simulink model "Solar_Batt_H2_PowerFlow_Solution_Lithium"  (R2023b)
settings: Solver=ode8  StartTime=0.0  StopTime=17520  FixedStep=1  RelTol=1e-3
values from neighbouring files (symbols this model uses):
  k1 = 0.6705    [main.m]
  n_batt = 40    [main.m]
  nb_set_solar_panel = 20    [main.m]
settings Model: Creator=pacel
settings DebuggingCC: UnconnectedInputMsg=warning  UnconnectedOutputMsg=warning  UnconnectedLineMsg=warning
settings ModelReferenceCC: EnableRefExpFcnMdlSchedulingChecks=on
settings RTWCC: DLArmComputeVersion=19.05

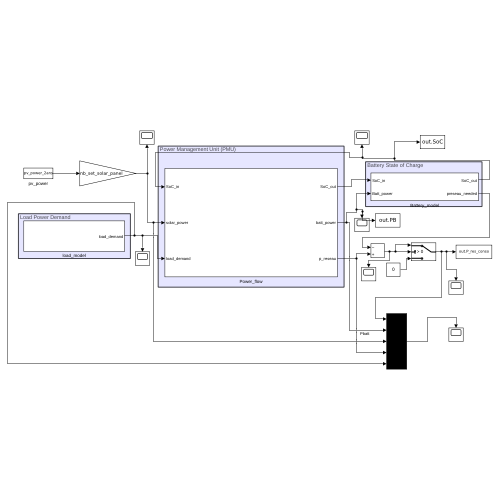
[thumbnail: Simulink's stored preview of the top-level diagram]
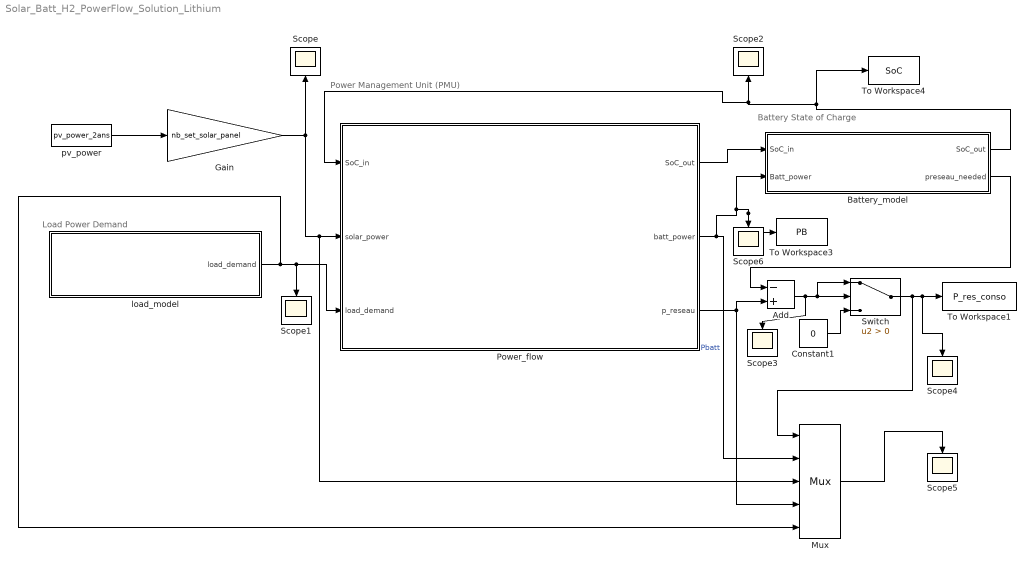
== system Solar_Batt_H2_PowerFlow_Solution_Lithium ==
  note: Load Power Demand
  note: Battery State of Charge
  note: Power Management Unit (PMU)
  Add : Sum  Inputs=-+
  Battery_model : Subsystem
  Constant1 : Constant  Value=0
  Gain : Gain  Gain=nb_set_solar_panel
  Mux : Mux  Inputs=5
  Power_flow : Subsystem
  Scope{,1..6} (7 alike) : Scope
  Switch : Switch  Criteria=u2 > Threshold  SaturateOnIntegerOverflow=off  InputSameDT=off
  To Workspace1 : ToWorkspace  VariableName=P_res_conso  SaveFormat=Timeseries  SampleTime=-1
  To Workspace3 : ToWorkspace  VariableName=PB  SaveFormat=Timeseries  SampleTime=-1
  To Workspace4 : ToWorkspace  VariableName=SoC  SaveFormat=Timeseries  SampleTime=-1
  load_model : Subsystem
  pv_power : FromWorkspace  VariableName=pv_power_2ans  OutDataTypeStr=double  SampleTime=1
  wires:
  Power_flow/2(batt_power) -> Battery_model/2(Batt_power), Scope6/1, To Workspace3/1, Mux/2  "Pbatt"
  load_model/1(load_demand) -> Mux/5, Scope1/1, Power_flow/3(load_demand)
  pv_power/1 -> Gain/1
  Battery_model/1(SoC_out) -> To Workspace4/1, Scope2/1, Power_flow/1(SoC_in)
  Power_flow/1(SoC_out) -> Battery_model/1(SoC_in)
  Gain/1 -> Scope/1, Mux/3, Power_flow/2(solar_power)
  Constant1/1 -> Switch/3
  Switch/1 -> Mux/1, Scope4/1, To Workspace1/1
  Mux/1 -> Scope5/1
  Power_flow/3(p_reseau) -> Mux/4, Add/2
  Battery_model/2(preseau_needed) -> Add/1
  Add/1 -> Scope3/1, Switch/2, Switch/1

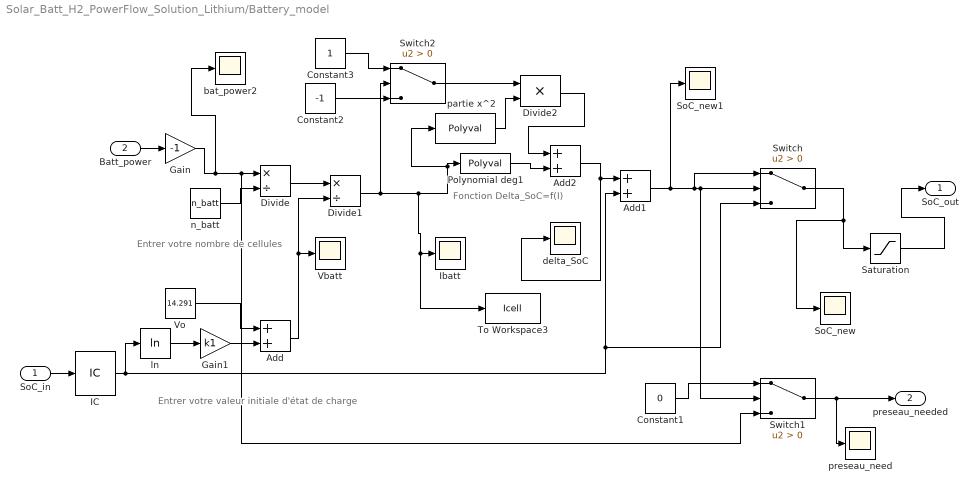
== system Solar_Batt_H2_PowerFlow_Solution_Lithium/Battery_model ==
  note: Entrer votre valeur initiale d'état de charge
  note: Entrer votre nombre de cellules
  note: Fonction Delta_SoC=f(I)
  SoC_in : Inport
  Batt_power : Inport  Port=2
  Add : Sum
  Add1 : Sum
  Add2 : Sum
  Constant1 : Constant  Value=0
  Constant2 : Constant  Value=-1
  Constant3 : Constant
  Divide : Product  Inputs=*/
  Divide1 : Product  Inputs=*/
  Divide2 : Product  Inputs=**
  Gain : Gain  Gain=-1
  Gain1 : Gain  Gain=k1
  IC : InitialCondition  Value=0.5
  Ibatt : Scope
  Polynomial deg1 : Polyval  Coefs=[ +0.01, -0.004 ]
  Saturation : Saturate  UpperLimit=0.95  LowerLimit=0.05
  SoC_new : Scope
  SoC_new1 : Scope
  Switch : Switch  Criteria=u2 > Threshold  SaturateOnIntegerOverflow=off  InputSameDT=off
  Switch1 : Switch  Criteria=u2 > Threshold  SaturateOnIntegerOverflow=off  InputSameDT=off
  Switch2 : Switch  Criteria=u2 > Threshold  SaturateOnIntegerOverflow=off  InputSameDT=off
  To Workspace3 : ToWorkspace  VariableName=Icell  SaveFormat=Timeseries  SampleTime=-1
  Vbatt : Scope
  Vo : Constant  Value=14.291
  bat_power2 : Scope
  delta_SoC : Scope
  ln : Math  Operator=log
  n_batt : Constant  Value=n_batt
  partie x^2 : Polyval  Coefs=[ 0, 0, 0]
  preseau_need : Scope
  SoC_out : Outport
  preseau_needed : Outport  Port=2
  wires:
  Saturation/1 -> SoC_out/1
  Batt_power/1 -> Gain/1
  Add/1 -> Divide1/2, Vbatt/1
  SoC_in/1 -> IC/1
  Vo/1 -> Add/1
  Divide1/1 -> Switch2/2, partie x^2/1, Polynomial deg1/1, To Workspace3/1, Ibatt/1
  Divide/1 -> Divide1/1
  Polynomial deg1/1 -> Add2/2
  n_batt/1 -> Divide/2
  Gain/1 -> bat_power2/1, Switch1/3, Divide/1
  Gain1/1 -> Add/2
  Switch/1 -> SoC_new/1, Saturation/1
  Add1/1 -> SoC_new1/1, Switch1/2, Switch/2, Switch/1
  Constant1/1 -> Switch1/1
  Switch1/1 -> preseau_need/1, preseau_needed/1
  Constant3/1 -> Switch2/1
  Constant2/1 -> Switch2/3
  Switch2/1 -> Divide2/1
  partie x^2/1 -> Divide2/2
  Divide2/1 -> Add2/1
  Add2/1 -> delta_SoC/1, Add1/1
  IC/1 -> ln/1, Switch/3, Add1/2
  ln/1 -> Gain1/1

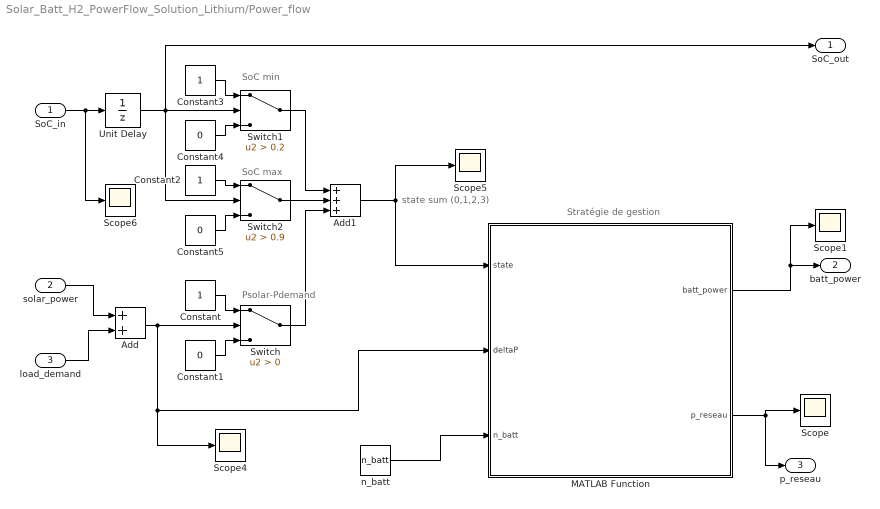
== system Solar_Batt_H2_PowerFlow_Solution_Lithium/Power_flow ==
  note: SoC min
  note: SoC max
  note: Psolar-Pdemand
  note: Stratégie de gestion
  note: state sum (0,1,2,3)
  SoC_in : Inport
  solar_power : Inport  Port=2
  load_demand : Inport  Port=3
  Add : Sum
  Add1 : Sum  Inputs=+++
  Constant : Constant
  Constant1 : Constant  Value=0
  Constant2 : Constant
  Constant3 : Constant
  Constant4 : Constant  Value=0
  Constant5 : Constant  Value=0
  MATLAB Function : MATLAB Function  TreatAsAtomicUnit=on
  Scope{,1,4..6} (5 alike) : Scope
  Switch : Switch  Criteria=u2 > Threshold  SaturateOnIntegerOverflow=off  InputSameDT=off
  Switch1 : Switch  Criteria=u2 > Threshold  Threshold=0.2  SaturateOnIntegerOverflow=off  InputSameDT=off
  Switch2 : Switch  Criteria=u2 > Threshold  Threshold=0.9  SaturateOnIntegerOverflow=off  InputSameDT=off
  Unit Delay : UnitDelay  SampleTime=-1  HasFrameUpgradeWarning=on
  n_batt : Constant  Value=n_batt
  SoC_out : Outport
  batt_power : Outport  Port=2
  p_reseau : Outport  Port=3
  wires:
  Unit Delay/1 -> SoC_out/1, Switch2/2, Switch1/2
  solar_power/1 -> Add/1
  Add1/1 -> MATLAB Function/1(state), Scope5/1
  Constant3/1 -> Switch1/1
  SoC_in/1 -> Scope6/1, Unit Delay/1
  Constant/1 -> Switch/1
  Constant1/1 -> Switch/3
  load_demand/1 -> Add/2
  Constant4/1 -> Switch1/3
  MATLAB Function/1(batt_power) -> batt_power/1, Scope1/1
  Constant2/1 -> Switch2/1
  Constant5/1 -> Switch2/3
  Switch2/1 -> Add1/2
  Add/1 -> Scope4/1, MATLAB Function/2(deltaP), Switch/2
  Switch1/1 -> Add1/1
  Switch/1 -> Add1/3
  MATLAB Function/2(p_reseau) -> Scope/1, p_reseau/1
  n_batt/1 -> MATLAB Function/3(n_batt)

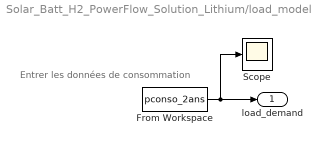
== system Solar_Batt_H2_PowerFlow_Solution_Lithium/load_model ==
  note: Entrer les données de consommation
  From Workspace : FromWorkspace  VariableName=pconso_2ans  OutDataTypeStr=double  SampleTime=1
  Scope : Scope
  load_demand : Outport
  wires:
  From Workspace/1 -> load_demand/1, Scope/1

== matlab function Solar_Batt_H2_PowerFlow_Solution_Lithium/Power_flow/MATLAB Function ==
  data: state input; batt_power output; deltaP input; p_reseau output; n_batt input
function [batt_power,p_reseau] = fcn(state,deltaP, n_batt)
if n_batt==0
    p_reseau=-deltaP;
    batt_power=0;
else
    if state==0 | state ==3 
        p_reseau= -deltaP;
        batt_power=0;
    else
        batt_power= -deltaP;
        p_reseau=0;
    end
end
